simulink model "M_PSK"  (Simulink 8.1)
settings: Solver=ode45  StartTime=0.0  StopTime=10.0  RelTol=1e-3
undefined symbols (not defined in the file): get, i
libraries: commdigbbndam3 x2, commviewers2 x2, commchan3 x1, commsink2 x1, commrandsrc2 x1
settings Model: Creator=Ammar  LastModifiedBy=User

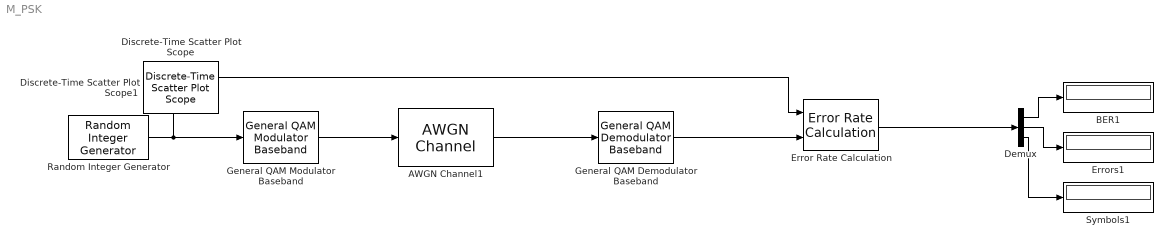
== system M_PSK ==
  AWGN Channel1 : commchan3/AWGN Channel  InputProcessing=Columns as channels (frame based)  seed=67  noiseMode="Signal to noise ratio  (Eb/No)"  EbNodB=3  EsNodB=6  SNRdB=10  bitsPerSym=3  Ps=1  Tsym=1/1000  variance=1
  BER1 : Display
  Demux : Demux  Outputs=3
  Error Rate Calculation : commsink2/Error Rate Calculation  N=0  st_delay=0  cp_mode=Entire frame  subframe=[]  PMode=Port  WsName=ErrorVec  RsMode2=off  stop=off  numErr=100  maxBits=1e6
  Errors1 : Display
  General QAM Demodulator Baseband : commdigbbndam3/General QAM Demodulator Baseband  SigCon=[exp(2*pi*i*[0:7]/8)]  OutType=Integer  DecType=Hard decision  VarSource=Dialog  Variance=1  outDtypeBit=Inherit via internal rule  outDtype=Inherit via internal rule  roundingMode=Floor  overflowMode=Wrap  sigConstWordLen=16  accum1WordLen=32  accum1FracLen=30  prodInWordLen=32  prodInFracLen=30  prodOutWordLen=32  prodOutFracLen=30  accum2WordLen=32  accum2FracLen=30  accum3WordLen=32  accum3FracLen=30  nsiWordLen=32  nsiFracLen=30  invn0WordLen=16  invn0FracLen=8  outputWordLen=32  outputFracLen=30
  General QAM Modulator Baseband : commdigbbndam3/General QAM Modulator Baseband  SigCon=[exp(2*pi*i*[0:7]/8)]  outDtype=double  outWordLen=16  outUDDataType=sfix(16)  outFracLenMode=Best precision  outFracLen=15
  Random Integer Generator : commrandsrc2/Random Integer Generator  mul=8  seed=35  Ts=1/1000  frameBased=off  sampPerFrame=1  orient=off  outDataType=double
  Symbols1 : Display
  Discrete-Time Scatter Plot Scope : commviewers2/Discrete-Time Scatter Plot Scope  Tag=ScatterPlot  IOType=viewer  sampPerSymb=1  offsetEye=0  numTraces=40  numNewFrames=10  LineMarkers=.  LineColors=b  fading=on  render=on  AxisGrid=on  xMin=-1.5  xMax=1.5  yMin=-1.5  yMax=1.5  inphaseLabel=In-phase Amplitude  quadratureLabel=Quadrature Amplitude  openScopeAtSimStart=on  FrameNumber=off  FigPos=get(0,'defaultfigureposition');  figTitle=Scatter Plot  numLinesMax=8  block_type_=scatter
  Discrete-Time Scatter Plot Scope1 : commviewers2/Discrete-Time Scatter Plot Scope  Tag=ScatterPlot  IOType=viewer  sampPerSymb=1  offsetEye=0  numTraces=40  numNewFrames=10  LineMarkers=.  LineColors=b  fading=on  render=on  AxisGrid=on  xMin=-1.5  xMax=1.5  yMin=-1.5  yMax=1.5  inphaseLabel=In-phase Amplitude  quadratureLabel=Quadrature Amplitude  openScopeAtSimStart=on  FrameNumber=off  FigPos=get(0,'defaultfigureposition');  figTitle=Scatter Plot  numLinesMax=8  block_type_=scatter
  wires:
  Random Integer Generator/1 -> General QAM Modulator Baseband/1, Error Rate Calculation/1
  Demux/1 -> BER1/1
  Demux/2 -> Errors1/1
  Demux/3 -> Symbols1/1
  Error Rate Calculation/1 -> Demux/1
  General QAM Modulator Baseband/1 -> AWGN Channel1/1
  AWGN Channel1/1 -> General QAM Demodulator Baseband/1
  General QAM Demodulator Baseband/1 -> Error Rate Calculation/2
